simulink model "cartesianLinearGuffanti"  (R2023a)
settings: Solver=ode4  StartTime=0.0  StopTime=10.0  FixedStep=dt  RelTol=1e-3
settings Model: Creator=ndelurgio  LastModifiedBy=ndelurgio

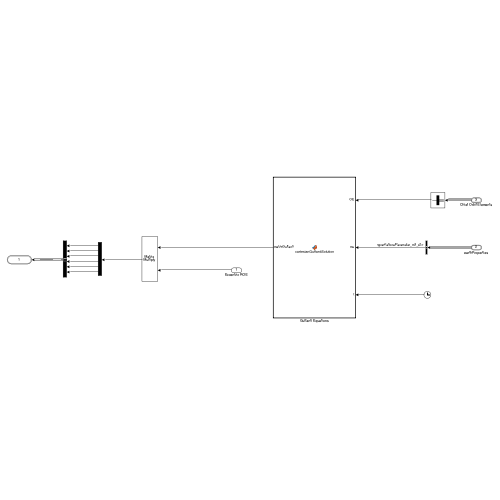
[thumbnail: Simulink's stored preview of the top-level diagram]
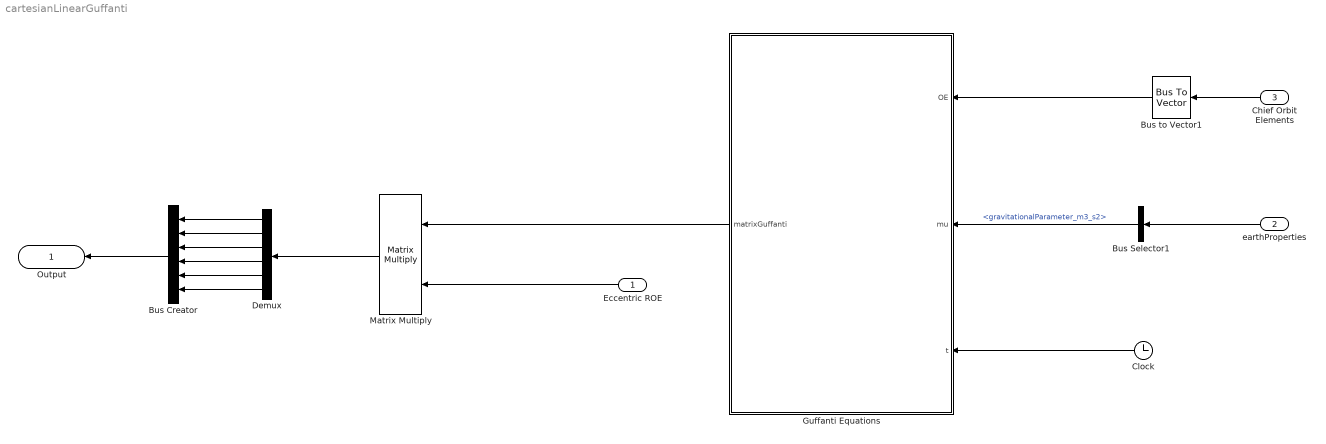
== system cartesianLinearGuffanti ==
  Eccentric ROE : Inport
  earthProperties : Inport  Port=2  OutDataTypeStr=Bus: earthProperties
  Chief Orbit Elements : Inport  Port=3  OutDataTypeStr=Bus: meanOrbitElements
  Bus Creator : BusCreator  Inputs=6  OutDataTypeStr=Bus: relativeCartesianState  NonVirtualBus=on
      settings: InheritFromInputs=off
  Bus Selector1 : BusSelector  OutputSignals=gravitationalParameter_m3_s2
  Bus to Vector1 : BusToVector
  Clock : Clock
  Demux : Demux  Outputs=6
  Guffanti Equations : MATLAB Function  TreatAsAtomicUnit=on
  Matrix Multiply : Product  Multiplication=Matrix(*)
  Output : Outport  OutDataTypeStr=Bus: relativeCartesianState
  wires:
  Chief Orbit Elements/1 -> Bus to Vector1/1
  earthProperties/1 -> Bus Selector1/1
  Bus Selector1/1 -> Guffanti Equations/2(mu)  "<gravitationalParameter_m3_s2>"
  Clock/1 -> Guffanti Equations/3(t)
  Guffanti Equations/1(matrixGuffanti) -> Matrix Multiply/1
  Demux/1 -> Bus Creator/1
  Demux/2 -> Bus Creator/2
  Demux/3 -> Bus Creator/3
  Demux/4 -> Bus Creator/4
  Demux/5 -> Bus Creator/5
  Demux/6 -> Bus Creator/6
  Bus Creator/1 -> Output/1
  Matrix Multiply/1 -> Demux/1
  Eccentric ROE/1 -> Matrix Multiply/2
  Bus to Vector1/1 -> Guffanti Equations/1(OE)

== matlab function cartesianLinearGuffanti/Guffanti Equations ==
  data: matrixGuffanti output; OE input; mu input; t input
function matrixGuffanti = cartesianGuffantiSolution(OE, mu, t)

matrixGuffanti = cartesianGuffantiSolution(OE, t, mu);

end
